simulink model "Copy_of_Five_Level"  (Simulink 8.4)
settings: Solver=ode45  StartTime=0.0  StopTime=1  RelTol=1e-3
undefined symbols (not defined in the file or in its folder): C, Cf1, Cf2, L, Lm, Lr, p, R, Rc1, Rc2, Rdc1, Rdc2, Rdc3, Rr, Tc, Ts, Uc_init
libraries: powerlib x106, simulink x3
settings Model: Creator=wangkui02  LastModifiedBy=Administrator-

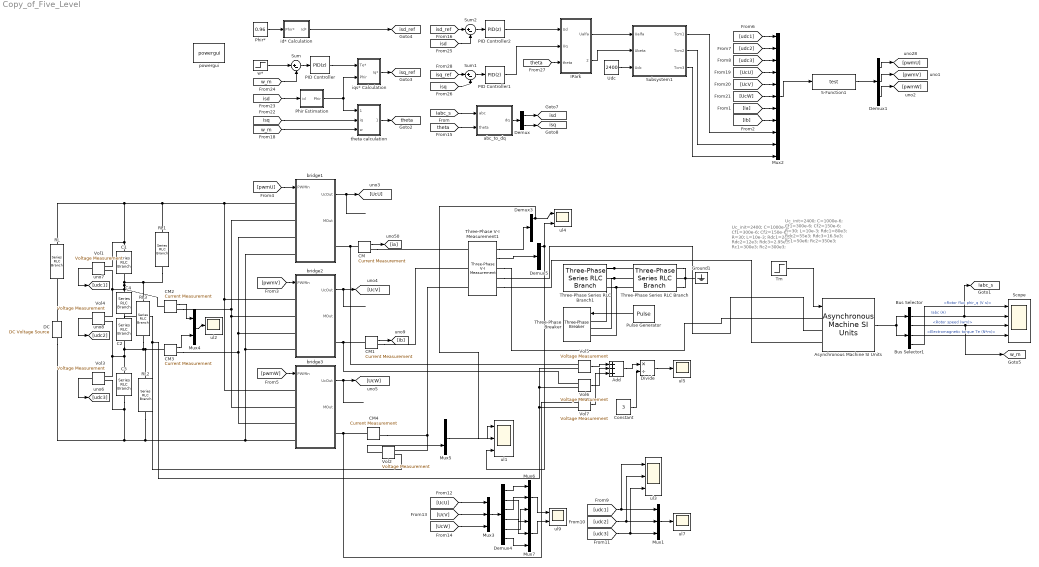
== system Copy_of_Five_Level ==
  note: Uc_init=2400;
      | C=1000e-6;
      | Cf1=300e-6;
      | Cf2=150e-6;
      | R=30;
      | L=10e-3;
      | Rdc1=2e6;
      | Rdc2=12e3;
      | Rdc3=2.95e3;
      | Rc1=300e3;
      | Rc2=300e3;
  note: Uc_init=2400;
      | C=1000e-6;
      | Cf1=300e-6;
      | Cf2=150e-6;
      | R=30;
      | L=10e-3;
      | Rdc1=80e3;
      | Rdc2=55e3;
      | Rdc3=16.5e3;
      | Rc1=50e6;
      | Rc2=350e3;
  Add : Sum  Inputs=+++
  Asynchronous Machine SI Units : powerlib/Machines/Asynchronous Machine SI Units  PresetModel=No  MechanicalLoad=Torque Tm  ShowDetailedParameters=on  RotorType=Squirrel-cage  ReferenceFrame=Stationary  Units=SI  MeasurementBus=off  NominalParameters=[2200 380 50]  Stator=[2.74 0.0138]  Rotor=[2.54 0.0138]  Cage1=[ 0.022 0.226/377]  Cage2=[ 0.022 0.226/377]  Lm=0.299  Mechanical=[0.0131 0.002985 2]  PolePairs=2  InitialConditions="[ 1,0   0,0,0   0,0,0 ]"  SimulateSaturation=off  Saturation=[14.03593122, 27.81365428, 53.79336849, 72.68890987, 97.98006896, 148.6815601, 215.7428561, 302.9841135, 428.7778367 ; 230, 322, 414, 460, 506, 552, 598, 644, 690]  LoadFlowParameters=0  TsPowergui=0  TsBlock=-1  IterativeModel=Forward Euler  Pmec=0
  Bus Selector : BusSelector  OutputSignals=Stator measurements.Stator current is_a (A),Stator measurements.Stator current is_b (A),Stator measurements.Stator current is_c (A)  OutputAsBus=on
  Bus Selector1 : BusSelector  OutputSignals=Mechanical.Rotor speed (wm),Mechanical.Electromagnetic torque Te (N*m),Rotor measurements.Rotor flux phir_q (V s)
  C1 : powerlib/Elements/Series RLC Branch  LConnTagsString=__new0  RConnTagsString=__new0  BranchType=C  Resistance=0.01  Inductance=1e-3  SetiL0=off  InitialCurrent=0  Capacitance=C  Setx0=on  InitialVoltage=Uc_init*1  Measurements=None
  C2 : powerlib/Elements/Series RLC Branch  LConnTagsString=__new0  RConnTagsString=__new0  BranchType=C  Resistance=0.01  Inductance=1e-3  SetiL0=off  InitialCurrent=0  Capacitance=C  Setx0=on  InitialVoltage=Uc_init  Measurements=None
  C3 : powerlib/Elements/Series RLC Branch  LConnTagsString=__new0  RConnTagsString=__new0  BranchType=C  Resistance=0.01  Inductance=1e-3  SetiL0=off  InitialCurrent=0  Capacitance=C*1  Setx0=on  InitialVoltage=Uc_init*1  Measurements=None
  C4 : powerlib/Elements/Series RLC Branch  LConnTagsString=__new0  RConnTagsString=__new0  BranchType=C  Resistance=0.01  Inductance=1e-3  SetiL0=off  InitialCurrent=0  Capacitance=C  Setx0=on  InitialVoltage=Uc_init  Measurements=None
  CM{,1..4} (5 alike) : powerlib/Measurements/Current Measurement  PhasorSimulation=off  OutputType=Complex  PSBequivalent=0
  Constant : Constant  Value=3
  DC : powerlib/Electrical Sources/DC Voltage Source  Amplitude=Uc_init*4  Measurements=None
  Demux : Demux  Outputs=2
  Demux1 : Demux  Outputs=[10 10 10]
  Demux3 : Demux  Outputs=3
  Demux4 : Demux  Outputs=6
  Demux5 : Demux  Outputs=3
  Divide : Product  Inputs=*/
  Ground1 : powerlib/Elements/Ground  LConnTagsString=a
  IPark : Subsystem
  Mux1 : Mux  Inputs=3
  Mux2 : Mux  Inputs=[1 1 1 2 2 2 1 1 1 1 1]
  Mux3 : Mux  Inputs=[2 2 2]
  Mux4 : Mux  Inputs=2
  Mux5 : Mux  Inputs=2
  Mux6 : Mux  Inputs=3
  Mux7 : Mux  Inputs=3
  PID Controller : simulink/Continuous/PID Controller  Controller=PID  TimeDomain=Discrete-time  SampleTime=Tc  IntegratorMethod=Forward Euler  FilterMethod=Forward Euler  Form=Parallel  P=0.075  I=10  D=0  N=100  InitialConditionSource=internal  InitialConditionForIntegrator=0  InitialConditionForFilter=0  ExternalReset=none  LimitOutput=on  UpperSaturationLimit=20  LowerSaturationLimit=-20  LinearizeAsGain=on  AntiWindupMode=none  Kb=1  TrackingMode=off  Kt=1  PParamMin=[]  PParamMax=[]  IParamMin=[]  IParamMax=[]  DParamMin=[]  DParamMax=[]  NParamMin=[]  NParamMax=[]  KbParamMin=[]  KbParamMax=[]  KtParamMin=[]  KtParamMax=[]  POutMin=[]  POutMax=[]  IOutMin=[]  IOutMax=[]  DOutMin=[]  DOutMax=[]  NOutMin=[]  NOutMax=[]  KbOutMin=[]  KbOutMax=[]  KtOutMin=[]  KtOutMax=[]  IntegratorOutMin=[]  IntegratorOutMax=[]  FilterOutMin=[]  FilterOutMax=[]  SumOutMin=[]  SumOutMax=[]  SumI1OutMin=[]  SumI1OutMax=[]  SumI2OutMin=[]  SumI2OutMax=[]  SumI3OutMin=[]  SumI3OutMax=[]  SumDOutMin=[]  SumDOutMax=[]  SaturationOutMin=[]  SaturationOutMax=[]  IntegratorContinuousStateAttributes=''  IntegratorStateMustResolveToSignalObject=off  IntegratorRTWStateStorageClass=Auto  FilterContinuousStateAttributes=''  FilterStateMustResolveToSignalObject=off  FilterRTWStateStorageClass=Auto  DifferentiatorICPrevScaledInput=0  DifferentiatorOutMin=[]  DifferentiatorOutMax=[]  UseFilter=on
  PID Controller1 : simulink/Continuous/PID Controller  Controller=PID  TimeDomain=Discrete-time  SampleTime=Tc  IntegratorMethod=Forward Euler  FilterMethod=Forward Euler  Form=Parallel  P=20  I=200  D=0  N=100  InitialConditionSource=internal  InitialConditionForIntegrator=0  InitialConditionForFilter=0  ExternalReset=none  LimitOutput=on  UpperSaturationLimit=500  LowerSaturationLimit=-500  LinearizeAsGain=on  AntiWindupMode=none  Kb=1  TrackingMode=off  Kt=1  PParamMin=[]  PParamMax=[]  IParamMin=[]  IParamMax=[]  DParamMin=[]  DParamMax=[]  NParamMin=[]  NParamMax=[]  KbParamMin=[]  KbParamMax=[]  KtParamMin=[]  KtParamMax=[]  POutMin=[]  POutMax=[]  IOutMin=[]  IOutMax=[]  DOutMin=[]  DOutMax=[]  NOutMin=[]  NOutMax=[]  KbOutMin=[]  KbOutMax=[]  KtOutMin=[]  KtOutMax=[]  IntegratorOutMin=[]  IntegratorOutMax=[]  FilterOutMin=[]  FilterOutMax=[]  SumOutMin=[]  SumOutMax=[]  SumI1OutMin=[]  SumI1OutMax=[]  SumI2OutMin=[]  SumI2OutMax=[]  SumI3OutMin=[]  SumI3OutMax=[]  SumDOutMin=[]  SumDOutMax=[]  SaturationOutMin=[]  SaturationOutMax=[]  IntegratorContinuousStateAttributes=''  IntegratorStateMustResolveToSignalObject=off  IntegratorRTWStateStorageClass=Auto  FilterContinuousStateAttributes=''  FilterStateMustResolveToSignalObject=off  FilterRTWStateStorageClass=Auto  DifferentiatorICPrevScaledInput=0  DifferentiatorOutMin=[]  DifferentiatorOutMax=[]  UseFilter=on
  PID Controller2 : simulink/Continuous/PID Controller  Controller=PID  TimeDomain=Discrete-time  SampleTime=Tc  IntegratorMethod=Forward Euler  FilterMethod=Forward Euler  Form=Parallel  P=20  I=200  D=0  N=100  InitialConditionSource=internal  InitialConditionForIntegrator=0  InitialConditionForFilter=0  ExternalReset=none  LimitOutput=on  UpperSaturationLimit=500  LowerSaturationLimit=-500  LinearizeAsGain=on  AntiWindupMode=none  Kb=1  TrackingMode=off  Kt=1  PParamMin=[]  PParamMax=[]  IParamMin=[]  IParamMax=[]  DParamMin=[]  DParamMax=[]  NParamMin=[]  NParamMax=[]  KbParamMin=[]  KbParamMax=[]  KtParamMin=[]  KtParamMax=[]  POutMin=[]  POutMax=[]  IOutMin=[]  IOutMax=[]  DOutMin=[]  DOutMax=[]  NOutMin=[]  NOutMax=[]  KbOutMin=[]  KbOutMax=[]  KtOutMin=[]  KtOutMax=[]  IntegratorOutMin=[]  IntegratorOutMax=[]  FilterOutMin=[]  FilterOutMax=[]  SumOutMin=[]  SumOutMax=[]  SumI1OutMin=[]  SumI1OutMax=[]  SumI2OutMin=[]  SumI2OutMax=[]  SumI3OutMin=[]  SumI3OutMax=[]  SumDOutMin=[]  SumDOutMax=[]  SaturationOutMin=[]  SaturationOutMax=[]  IntegratorContinuousStateAttributes=''  IntegratorStateMustResolveToSignalObject=off  IntegratorRTWStateStorageClass=Auto  FilterContinuousStateAttributes=''  FilterStateMustResolveToSignalObject=off  FilterRTWStateStorageClass=Auto  DifferentiatorICPrevScaledInput=0  DifferentiatorOutMin=[]  DifferentiatorOutMax=[]  UseFilter=on
  Phir Estimation : Subsystem
  Phir* : Constant  Value=0.96
  Pulse Generator : DiscretePulseGenerator  PulseType=Time based  PulseWidth=50
  RL : powerlib/Elements/Series RLC Branch  LConnTagsString=__new0  RConnTagsString=__new0  BranchType=RL  Resistance=0.01  Inductance=1e-6  SetiL0=off  InitialCurrent=0  Capacitance=1e-6  Setx0=off  InitialVoltage=0  Measurements=None
  RL1 : powerlib/Elements/Series RLC Branch  LConnTagsString=__new0  RConnTagsString=__new0  BranchType=R  Resistance=Rdc1  Inductance=1e-6  SetiL0=off  InitialCurrent=0  Capacitance=1e-6  Setx0=off  InitialVoltage=0  Measurements=None
  RL2 : powerlib/Elements/Series RLC Branch  LConnTagsString=__new0  RConnTagsString=__new0  BranchType=R  Resistance=Rdc3  Inductance=1e-6  SetiL0=off  InitialCurrent=0  Capacitance=1e-6  Setx0=off  InitialVoltage=0  Measurements=None
  RL3 : powerlib/Elements/Series RLC Branch  LConnTagsString=__new0  RConnTagsString=__new0  BranchType=R  Resistance=Rdc2  Inductance=1e-6  SetiL0=off  InitialCurrent=0  Capacitance=1e-6  Setx0=off  InitialVoltage=0  Measurements=None
  S-Function1 : S-Function  FunctionName=test  EnableBusSupport=off
  Scope : Scope  NumInputPorts=4
      settings: YMin=-0.1~-40~-20~-5  YMax=0.4~40~5~10  SaveName=ScopeData9  Decimation=20  SampleTime=5e-6
  Subsystem1 : Subsystem
  Sum : Sum  Inputs=|+-
  Sum1 : Sum  Inputs=|+-
  Sum2 : Sum  Inputs=|+-
  Three-Phase Series RLC Branch : powerlib/Elements/Three-Phase Series RLC Branch  LConnTagsString=A|B|C  RConnTagsString=A|B|C  BranchType=RL  Resistance=R  Inductance=L  Capacitance=1e-6  Measurements=Branch voltages and currents
  Three-Phase Series RLC Branch1 : powerlib/Elements/Three-Phase Series RLC Branch  LConnTagsString=A|B|C  RConnTagsString=A|B|C  BranchType=RL  Resistance=R  Inductance=L  Capacitance=1e-6  Measurements=Branch voltages and currents
  Three-Phase V-I Measurement1 : powerlib/Measurements/Three-Phase V-I Measurement  VoltageMeasurement=phase-to-phase  SetLabelV=off  LabelV=Vabc  Vpu=off  VpuLL=off  CurrentMeasurement=yes  SetLabelI=off  LabelI=Iabc  Ipu=off  Pbase=100e6  Vbase=500e3  OutputType=Complex  PhasorSimulation=off  PSBequivalent=0
  Three-Phase Breaker : powerlib/Elements/Three-Phase Breaker  InitialState=closed  SwitchA=on  SwitchB=on  SwitchC=on  SwitchTimes="[4/60  10/60]"  External=on  BreakerResistance=0.001  SnubberResistance=1e6  SnubberCapacitance=inf  Measurements=None
  Tm : Step  Time=0.1  After=5  SampleTime=0
  Udc : Constant  Value=2400
  Vol{1..7} (7 alike) : powerlib/Measurements/Voltage Measurement  PhasorSimulation=off  OutputType=Complex  PSBequivalent=0
  abc_to_dq : Subsystem
  bridge1 : Subsystem
  bridge2 : Subsystem
  bridge3 : Subsystem
  id* Calculation : Subsystem
  iqs* Calculation : Subsystem
  powergui : powerlib/powergui  Priority=1  SimulationMode=Discrete  SolverType=Tustin/Backward Euler (TBE)  SampleTime=Ts  frequency=60  SPID=off  DisableSnubberDevices=off  DisableRonSwitches=off  DisableVfSwitches=off  SwTol=0  DisplayEquations=off  Interpol=off  methode=off  Ts=10  frequencyindice=0  Pbase=100e6  ErrMax=1e-4  Iterations=50  UnitsV=kV  UnitsW=MW  FunctionMessages=off  echomessages=off  HookPort=off  EnableUseOfTLC=off  x0status=blocks  RestoreLinks=warning  ResistiveCurrentMeasurement=off  Frange=[0:2:500]  Ylog=off  Xlog=on  ShowGrid=off  save=off  variable=ZData  structure=0  ZoomFFT=off  StartTime=0.0  cycles=1  DisplayStyle=1  fundamental=60  FreqAxis=off  MaxFrequency=1000  frequencyindicesteady=1  RmsSteady=1  display=off
  theta calculation : Subsystem  mask{Lr=Lr, Lm=Lm, Rr=Rr}
  ul1 : Scope  NumInputPorts=3
      settings: YMin=-5000~-10000~-150  YMax=5000~10000~150  SaveName=io  MaxDataPoints=100000  Decimation=10
  ul2 : Scope
      settings: YMin=-200  YMax=200  SaveName=udc1  MaxDataPoints=100000  Decimation=10
  ul3 : Scope  NumInputPorts=3
      settings: TimeRange=1  YMin=2385~4780~2340  YMax=2405~4900~2400  SaveName=ucf1  MaxDataPoints=100000
  ul4 : Scope  NumInputPorts=2
      settings: YMin=-0.0025~-4  YMax=0.001~14  SaveName=ul  MaxDataPoints=100000  Decimation=10
  ul5 : Scope
      settings: TimeRange=1  YMin=-5000  YMax=-1500  SaveName=udc2  MaxDataPoints=100000  Decimation=10
  ul7 : Scope
      settings: YMin=2000  YMax=5000  SaveName=udc  MaxDataPoints=100000  Decimation=10
  ul9 : Scope  NumInputPorts=2
      settings: TimeRange=0.2  YMin=4500~2395  YMax=4850~2440  SaveName=ucf  MaxDataPoints=100000
  w* : Step  Time=0.01  After=1000/30*pi  SampleTime=0
  tag scope: Iabc_s=global, isd=global, isd_ref=global, isq=global, isq_ref=global, theta=global, w_m=global
  wires:
  bridge1/1(UcOut) -> [UcU]
  [pwmU] -> bridge1/1(PWMIn)
  [pwmV] -> bridge2/1(PWMIn)
  [pwmW] -> bridge3/1(PWMIn)
  Vol2/1 -> Mux5/2
  bridge2/1(UcOut) -> [UcV]
  Vol1/1 -> [udc1]
  Vol3/1 -> [udc3]
  bridge3/1(UcOut) -> [UcW]
  Vol4/1 -> [udc2]
  [udc1] -> Mux1/1, ul3/1
  [udc2] -> Mux1/2, ul3/2
  [udc3] -> Mux1/3, ul3/3
  Mux1/1 -> ul7/1
  Three-Phase V-I Measurement1/1 -> Demux3/1
  Demux3/1 -> ul4/1, ul1/2
  CM/1 -> [ia]
  CM1/1 -> [ib]
  [UcU] -> Mux3/1
  [UcV] -> Mux3/2
  [UcW] -> Mux3/3
  Pulse Generator/1 -> Three-Phase Breaker/1
  CM2/1 -> Mux4/1
  Mux4/1 -> ul2/1
  CM3/1 -> Mux4/2
  Mux5/1 -> ul1/1
  Mux3/1 -> Demux4/1
  Demux4/1 -> Mux6/1
  Demux4/3 -> Mux6/2
  Demux4/5 -> Mux6/3
  Demux4/2 -> Mux7/1
  Demux4/4 -> Mux7/2
  Mux6/1 -> ul9/1
  Mux7/1 -> ul9/2
  Demux4/6 -> Mux7/3
  Three-Phase V-I Measurement1/2 -> Demux5/1
  Demux5/1 -> ul4/2, ul1/3
  Vol5/1 -> Add/1
  Vol6/1 -> Add/2
  Vol7/1 -> Add/3
  Divide/1 -> ul5/1
  Add/1 -> Divide/1
  Constant/1 -> Divide/2
  [Iabc_s] -> abc_to_dq/1(abc)
  [theta] -> abc_to_dq/2(theta)
  abc_to_dq/1(dq) -> Demux/1
  Demux/1 -> [isd]
  Demux/2 -> [isq]
  Phir*/1 -> id* Calculation/1(Phir*)
  PID Controller/1 -> iqs* Calculation/1(Te*)
  [w_m] -> theta calculation/3(w)
  Phir Estimation/1(Phir) -> theta calculation/1(Phir), iqs* Calculation/2(Phir)
  [isq] -> theta calculation/2(iq)
  [isd] -> Phir Estimation/1(id)
  [w_m] -> Sum/2
  theta calculation/1(theta) -> [theta]
  [isd] -> Sum2/2
  PID Controller1/1 -> IPark/2(Uq)
  [theta] -> IPark/3(theta)
  Sum/1 -> PID Controller/1
  w*/1 -> Sum/1
  iqs* Calculation/1(Iq*) -> [isq_ref]
  Sum1/1 -> PID Controller1/1
  [isq_ref] -> Sum1/1
  [isq] -> Sum1/2
  id* Calculation/1(Id*) -> [isd_ref]
  [isd_ref] -> Sum2/1
  Sum2/1 -> PID Controller2/1
  PID Controller2/1 -> IPark/1(Ud)
  Udc/1 -> Subsystem1/3(Udc)
  IPark/1(Ualfa) -> Subsystem1/1(Ualfa)
  IPark/2(Ubeta) -> Subsystem1/2(Ubeta)
  Tm/1 -> Asynchronous Machine SI Units/1
  Subsystem1/1(Tcm1) -> Mux2/9
  Demux1/1 -> [pwmU]
  Demux1/2 -> [pwmV]
  Demux1/3 -> [pwmW]
  [udc1] -> Mux2/1
  [udc2] -> Mux2/2
  [UcU] -> Mux2/4
  [UcV] -> Mux2/5
  [UcW] -> Mux2/6
  [ia] -> Mux2/7
  [ib] -> Mux2/8
  [udc3] -> Mux2/3
  Subsystem1/2(Tcm2) -> Mux2/10
  Subsystem1/3(Tcm3) -> Mux2/11
  Bus Selector1/1 -> Scope/3, [w_m]  "<Rotor speed (wm)>"
  Bus Selector/1 -> [Iabc_s], Scope/2  "Iabc (A)"
  Bus Selector1/2 -> Scope/4  "<Electromagnetic torque Te (N*m)>"
  Asynchronous Machine SI Units/1 -> Bus Selector/1, Bus Selector1/1
  Bus Selector1/3 -> Scope/1  "<Rotor flux phir_q (V s)>"
  Mux2/1 -> S-Function1/1
  S-Function1/1 -> Demux1/1
  connections:
  Ground1/LConn1 -- Three-Phase Series RLC Branch/RConn2 -- Three-Phase Series RLC Branch/RConn1 -- Three-Phase Series RLC Branch/RConn3
  Three-Phase V-I Measurement1/LConn3 -- Vol2/LConn1 -- CM4/RConn1
  C1/LConn1 -- Vol1/LConn1 -- RL/LConn1 -- bridge3/LConn1 -- bridge2/LConn1 -- bridge1/LConn1 -- RL1/LConn1
  C3/RConn1 -- Vol3/LConn2 -- DC/LConn1 -- bridge3/LConn4 -- bridge1/LConn4 -- bridge2/LConn4 -- RL2/RConn1
  DC/RConn1 -- RL/RConn1
  bridge3/LConn3 -- bridge1/LConn3 -- bridge2/LConn3 -- CM3/RConn1
  CM2/RConn1 -- bridge3/LConn2 -- bridge2/LConn2 -- bridge1/LConn2
  CM/LConn1 -- Vol5/LConn1 -- bridge1/RConn1
  CM/RConn1 -- Three-Phase V-I Measurement1/LConn1
  bridge2/RConn1 -- Vol6/LConn1 -- CM1/LConn1
  CM1/RConn1 -- Three-Phase V-I Measurement1/LConn2
  Three-Phase V-I Measurement1/RConn1 -- Asynchronous Machine SI Units/LConn1
  Three-Phase Series RLC Branch1/RConn1 -- Three-Phase Breaker/LConn1 -- Three-Phase Series RLC Branch/LConn1
  Three-Phase Series RLC Branch1/RConn2 -- Three-Phase Breaker/LConn2 -- Three-Phase Series RLC Branch/LConn2
  Three-Phase Series RLC Branch1/RConn3 -- Three-Phase Series RLC Branch/LConn3 -- Three-Phase Breaker/LConn3
  RL1/RConn1 -- CM2/LConn1 -- Vol4/LConn1 -- Vol1/LConn2 -- C4/LConn1 -- C1/RConn1 -- RL3/LConn1
  CM3/LConn1 -- Vol4/LConn2 -- Vol3/LConn1 -- C3/LConn1 -- C2/RConn1 -- RL3/RConn1 -- RL2/LConn1
  CM4/LConn1 -- Vol7/LConn1 -- bridge3/RConn1
  C4/RConn1 -- Vol7/LConn2 -- Vol6/LConn2 -- Vol5/LConn2 -- Vol2/LConn2
  Three-Phase V-I Measurement1/RConn2 -- Asynchronous Machine SI Units/LConn2
  Three-Phase V-I Measurement1/RConn3 -- Asynchronous Machine SI Units/LConn3

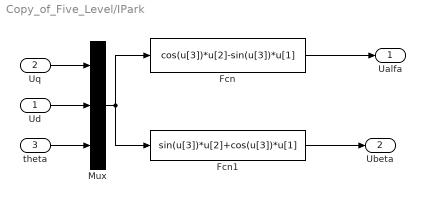
== system Copy_of_Five_Level/IPark ==
  Ud : Inport
  Uq : Inport  Port=2
  theta : Inport  Port=3
  Fcn : Fcn  Expr=cos(u[3])*u[2]-sin(u[3])*u[1]
  Fcn1 : Fcn  Expr=sin(u[3])*u[2]+cos(u[3])*u[1]
  Mux : Mux  Inputs=3
  Ualfa : Outport
  Ubeta : Outport  Port=2
  wires:
  Uq/1 -> Mux/1
  Ud/1 -> Mux/2
  theta/1 -> Mux/3
  Mux/1 -> Fcn/1, Fcn1/1
  Fcn/1 -> Ualfa/1
  Fcn1/1 -> Ubeta/1

== system Copy_of_Five_Level/Phir Estimation ==
  id : Inport
  Gain : Gain  Gain=Lm*Rr  SaturateOnIntegerOverflow=on  OutDataTypeStr=Inherit: Same as input  ParamDataTypeStr=Inherit: Same as input
  Transfer Fcn : TransferFcn  Denominator=[Lr Rr]
  Phir : Outport
  wires:
  Transfer Fcn/1 -> Phir/1
  Gain/1 -> Transfer Fcn/1
  id/1 -> Gain/1

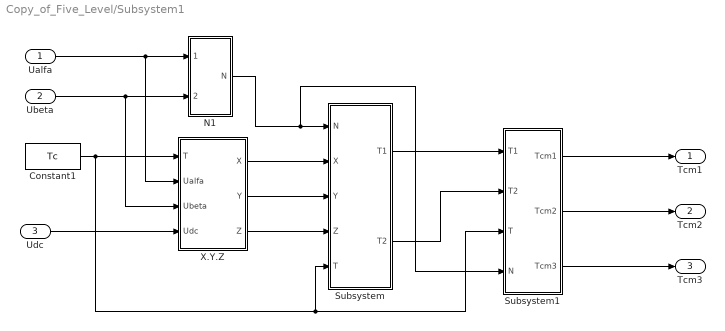
== system Copy_of_Five_Level/Subsystem1 ==
  Ualfa : Inport
  Ubeta : Inport  Port=2
  Udc : Inport  Port=3
  Constant1 : Constant  Value=Tc
  N1 : Subsystem
  Subsystem : Subsystem
  Subsystem1 : Subsystem
  X.Y.Z : Subsystem
  Tcm1 : Outport
  Tcm2 : Outport  Port=2
  Tcm3 : Outport  Port=3
  wires:
  Constant1/1 -> Subsystem1/3(T), Subsystem/5(T), X.Y.Z/1(T)
  X.Y.Z/1(X) -> Subsystem/2(X)
  X.Y.Z/2(Y) -> Subsystem/3(Y)
  X.Y.Z/3(Z) -> Subsystem/4(Z)
  Subsystem1/1(Tcm1) -> Tcm1/1
  Subsystem1/2(Tcm2) -> Tcm2/1
  Subsystem1/3(Tcm3) -> Tcm3/1
  Subsystem/1(T1) -> Subsystem1/1(T1)
  Subsystem/2(T2) -> Subsystem1/2(T2)
  N1/1(N) -> Subsystem/1(N), Subsystem1/4(N)
  Udc/1 -> X.Y.Z/4(Udc)
  Ualfa/1 -> X.Y.Z/2(Ualfa), N1/1(Ualfa)
  Ubeta/1 -> X.Y.Z/3(Ubeta), N1/2(Ubeta)

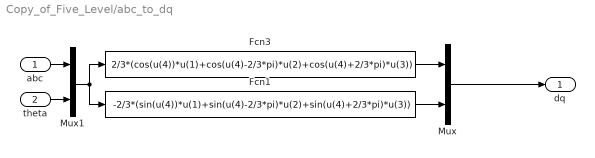
== system Copy_of_Five_Level/abc_to_dq ==
  abc : Inport
  theta : Inport  Port=2
  Fcn1 : Fcn  Expr=-2/3*(sin(u(4))*u(1)+sin(u(4)-2/3*pi)*u(2)+sin(u(4)+2/3*pi)*u(3))
  Fcn3 : Fcn  Expr=2/3*(cos(u(4))*u(1)+cos(u(4)-2/3*pi)*u(2)+cos(u(4)+2/3*pi)*u(3))
  Mux : Mux  Inputs=2
  Mux1 : Mux  Inputs=2
  dq : Outport
  wires:
  Fcn3/1 -> Mux/1
  Fcn1/1 -> Mux/2
  abc/1 -> Mux1/1
  theta/1 -> Mux1/2
  Mux1/1 -> Fcn3/1, Fcn1/1
  Mux/1 -> dq/1

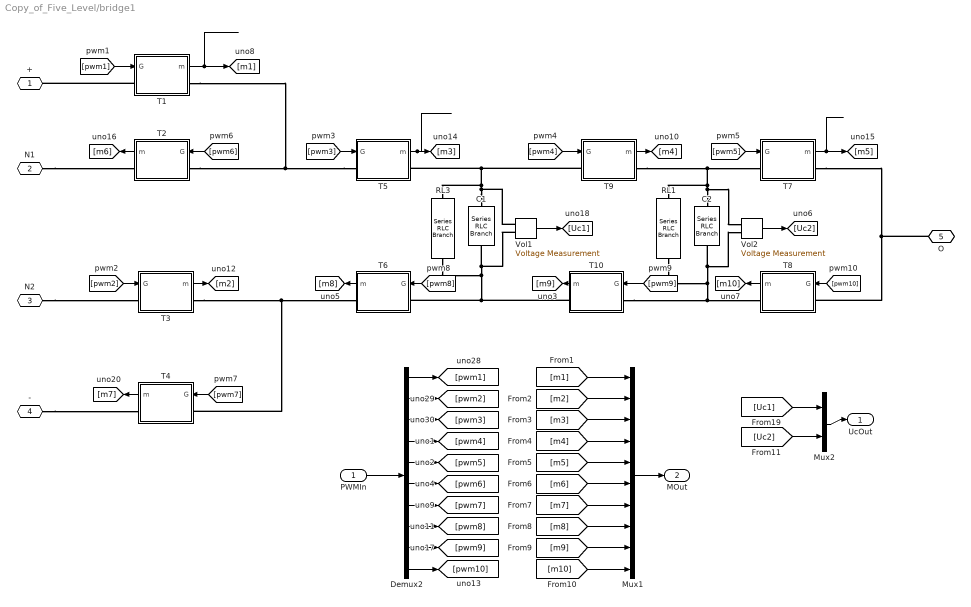
== system Copy_of_Five_Level/bridge1 ==
  PWMIn : Inport
  C1 : powerlib/Elements/Series RLC Branch  LConnTagsString=__new0  RConnTagsString=__new0  BranchType=C  Resistance=1  Inductance=1e-3  SetiL0=off  InitialCurrent=0  Capacitance=Cf2  Setx0=on  InitialVoltage=Uc_init*2*1  Measurements=None
  C2 : powerlib/Elements/Series RLC Branch  LConnTagsString=__new0  RConnTagsString=__new0  BranchType=C  Resistance=1  Inductance=1e-3  SetiL0=off  InitialCurrent=0  Capacitance=Cf1  Setx0=on  InitialVoltage=Uc_init*1  Measurements=None
  Demux2 : Demux  Outputs=10
  Mux1 : Mux  Inputs=10
  Mux2 : Mux  Inputs=2
  RL1 : powerlib/Elements/Series RLC Branch  LConnTagsString=__new0  RConnTagsString=__new0  BranchType=R  Resistance=Rc1  Inductance=1e-6  SetiL0=off  InitialCurrent=0  Capacitance=1e-6  Setx0=off  InitialVoltage=0  Measurements=None
  RL3 : powerlib/Elements/Series RLC Branch  LConnTagsString=__new0  RConnTagsString=__new0  BranchType=R  Resistance=Rc2  Inductance=1e-6  SetiL0=off  InitialCurrent=0  Capacitance=1e-6  Setx0=off  InitialVoltage=0  Measurements=None
  T1 : Subsystem
  T10 : Subsystem
  T2 : Subsystem
  T3 : Subsystem
  T4 : Subsystem
  T5 : Subsystem
  T6 : Subsystem
  T7 : Subsystem
  T8 : Subsystem
  T9 : Subsystem
  Vol1 : powerlib/Measurements/Voltage Measurement  PhasorSimulation=off  OutputType=Complex  PSBequivalent=0
  Vol2 : powerlib/Measurements/Voltage Measurement  PhasorSimulation=off  OutputType=Complex  PSBequivalent=0
  + : PMIOPort  Port=1  Side=Left
  N1 : PMIOPort  Port=2  Side=Left
  N2 : PMIOPort  Port=3  Side=Left
  - : PMIOPort  Port=4  Side=Left
  O : PMIOPort  Port=5  Side=Right
  UcOut : Outport
  MOut : Outport  Port=2
  wires:
  T1/1(m) -> [m1]
  [pwm2] -> T3/1(G)
  T3/1(m) -> [m2]
  [pwm3] -> T5/1(G)
  T5/1(m) -> [m3]
  [pwm5] -> T7/1(G)
  T7/1(m) -> [m5]
  [pwm6] -> T2/1(G)
  [pwm7] -> T4/1(G)
  T4/1(m) -> [m7]
  PWMIn/1 -> Demux2/1
  Demux2/1 -> [pwm1]
  Demux2/2 -> [pwm2]
  Demux2/3 -> [pwm3]
  Demux2/4 -> [pwm4]
  Demux2/5 -> [pwm5]
  Demux2/6 -> [pwm6]
  Demux2/7 -> [pwm7]
  Demux2/8 -> [pwm8]
  [pwm1] -> T1/1(G)
  T2/1(m) -> [m6]
  [m1] -> Mux1/1
  [m2] -> Mux1/2
  [m3] -> Mux1/3
  [m4] -> Mux1/4
  [m5] -> Mux1/5
  [m6] -> Mux1/6
  [m7] -> Mux1/7
  [m8] -> Mux1/8
  Mux1/1 -> MOut/1
  [pwm10] -> T8/1(G)
  T8/1(m) -> [m10]
  [pwm8] -> T6/1(G)
  T6/1(m) -> [m8]
  Vol2/1 -> [Uc2]
  [pwm4] -> T9/1(G)
  [pwm9] -> T10/1(G)
  T10/1(m) -> [m9]
  T9/1(m) -> [m4]
  Demux2/9 -> [pwm9]
  Demux2/10 -> [pwm10]
  [m9] -> Mux1/9
  [m10] -> Mux1/10
  Vol1/1 -> [Uc1]
  Mux2/1 -> UcOut/1
  [Uc1] -> Mux2/1
  [Uc2] -> Mux2/2
  connections:
  T1/LConn1 -- +/RConn1
  -/RConn1 -- T4/RConn1
  C2/RConn1 -- Vol2/LConn2 -- T10/LConn1 -- T8/RConn1 -- RL1/RConn1
  C2/LConn1 -- Vol2/LConn1 -- T7/LConn1 -- T9/RConn1 -- RL1/LConn1
  T8/LConn1 -- O/RConn1 -- T7/RConn1
  N1/RConn1 -- T2/RConn1
  N2/RConn1 -- T3/LConn1
  T5/LConn1 -- T1/RConn1 -- T2/LConn1
  T3/RConn1 -- T6/RConn1 -- T4/LConn1
  C1/RConn1 -- Vol1/LConn2 -- T10/RConn1 -- T6/LConn1 -- RL3/RConn1
  C1/LConn1 -- T9/LConn1 -- T5/RConn1 -- RL3/LConn1 -- Vol1/LConn1

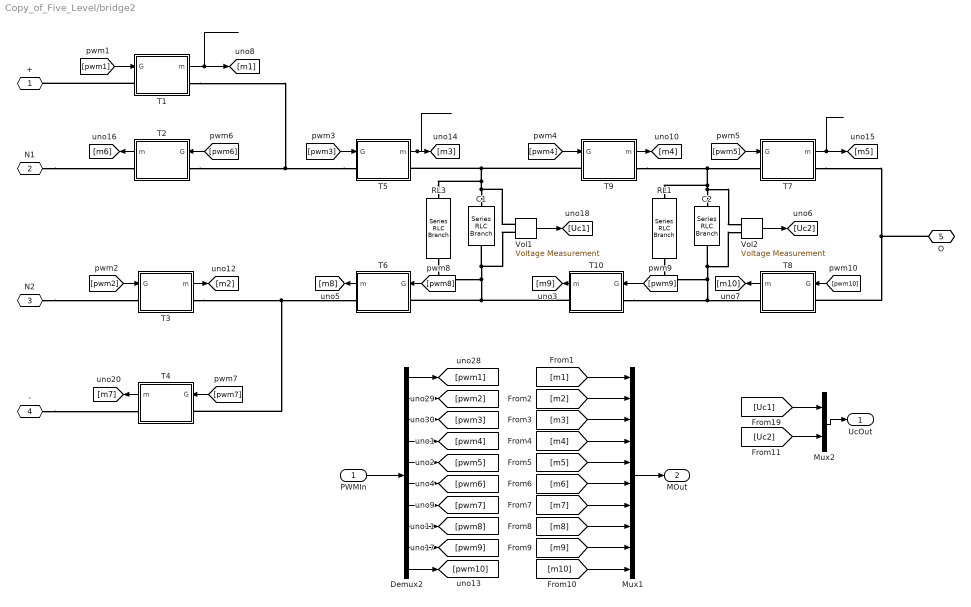
== system Copy_of_Five_Level/bridge2 ==
  PWMIn : Inport
  C1 : powerlib/Elements/Series RLC Branch  LConnTagsString=__new0  RConnTagsString=__new0  BranchType=C  Resistance=1  Inductance=1e-3  SetiL0=off  InitialCurrent=0  Capacitance=Cf2  Setx0=on  InitialVoltage=Uc_init*2  Measurements=None
  C2 : powerlib/Elements/Series RLC Branch  LConnTagsString=__new0  RConnTagsString=__new0  BranchType=C  Resistance=1  Inductance=1e-3  SetiL0=off  InitialCurrent=0  Capacitance=Cf1  Setx0=on  InitialVoltage=Uc_init  Measurements=None
  Demux2 : Demux  Outputs=10
  Mux1 : Mux  Inputs=10
  Mux2 : Mux  Inputs=2
  RL1 : powerlib/Elements/Series RLC Branch  LConnTagsString=__new0  RConnTagsString=__new0  BranchType=R  Resistance=Rc1  Inductance=1e-6  SetiL0=off  InitialCurrent=0  Capacitance=1e-6  Setx0=off  InitialVoltage=0  Measurements=None
  RL3 : powerlib/Elements/Series RLC Branch  LConnTagsString=__new0  RConnTagsString=__new0  BranchType=R  Resistance=Rc2  Inductance=1e-6  SetiL0=off  InitialCurrent=0  Capacitance=1e-6  Setx0=off  InitialVoltage=0  Measurements=None
  T1 : Subsystem
  T10 : Subsystem
  T2 : Subsystem
  T3 : Subsystem
  T4 : Subsystem
  T5 : Subsystem
  T6 : Subsystem
  T7 : Subsystem
  T8 : Subsystem
  T9 : Subsystem
  Vol1 : powerlib/Measurements/Voltage Measurement  PhasorSimulation=off  OutputType=Complex  PSBequivalent=0
  Vol2 : powerlib/Measurements/Voltage Measurement  PhasorSimulation=off  OutputType=Complex  PSBequivalent=0
  + : PMIOPort  Port=1  Side=Left
  N1 : PMIOPort  Port=2  Side=Left
  N2 : PMIOPort  Port=3  Side=Left
  - : PMIOPort  Port=4  Side=Left
  O : PMIOPort  Port=5  Side=Right
  UcOut : Outport
  MOut : Outport  Port=2
  wires:
  T1/1(m) -> [m1]
  [pwm2] -> T3/1(G)
  T3/1(m) -> [m2]
  [pwm3] -> T5/1(G)
  T5/1(m) -> [m3]
  [pwm5] -> T7/1(G)
  T7/1(m) -> [m5]
  [pwm6] -> T2/1(G)
  [pwm7] -> T4/1(G)
  T4/1(m) -> [m7]
  PWMIn/1 -> Demux2/1
  Demux2/1 -> [pwm1]
  Demux2/2 -> [pwm2]
  Demux2/3 -> [pwm3]
  Demux2/4 -> [pwm4]
  Demux2/5 -> [pwm5]
  Demux2/6 -> [pwm6]
  Demux2/7 -> [pwm7]
  Demux2/8 -> [pwm8]
  [pwm1] -> T1/1(G)
  T2/1(m) -> [m6]
  [m1] -> Mux1/1
  [m2] -> Mux1/2
  [m3] -> Mux1/3
  [m4] -> Mux1/4
  [m5] -> Mux1/5
  [m6] -> Mux1/6
  [m7] -> Mux1/7
  [m8] -> Mux1/8
  Mux1/1 -> MOut/1
  [pwm10] -> T8/1(G)
  T8/1(m) -> [m10]
  [pwm8] -> T6/1(G)
  T6/1(m) -> [m8]
  Vol2/1 -> [Uc2]
  [pwm4] -> T9/1(G)
  [pwm9] -> T10/1(G)
  T10/1(m) -> [m9]
  T9/1(m) -> [m4]
  Demux2/9 -> [pwm9]
  Demux2/10 -> [pwm10]
  [m9] -> Mux1/9
  [m10] -> Mux1/10
  Vol1/1 -> [Uc1]
  Mux2/1 -> UcOut/1
  [Uc1] -> Mux2/1
  [Uc2] -> Mux2/2
  connections:
  T1/LConn1 -- +/RConn1
  -/RConn1 -- T4/RConn1
  C2/RConn1 -- Vol2/LConn2 -- T10/LConn1 -- T8/RConn1 -- RL1/RConn1
  C2/LConn1 -- Vol2/LConn1 -- T7/LConn1 -- T9/RConn1 -- RL1/LConn1
  T8/LConn1 -- O/RConn1 -- T7/RConn1
  N1/RConn1 -- T2/RConn1
  N2/RConn1 -- T3/LConn1
  T5/LConn1 -- T1/RConn1 -- T2/LConn1
  T3/RConn1 -- T6/RConn1 -- T4/LConn1
  RL3/RConn1 -- C1/RConn1 -- Vol1/LConn2 -- T10/RConn1 -- T6/LConn1
  RL3/LConn1 -- C1/LConn1 -- Vol1/LConn1 -- T9/LConn1 -- T5/RConn1

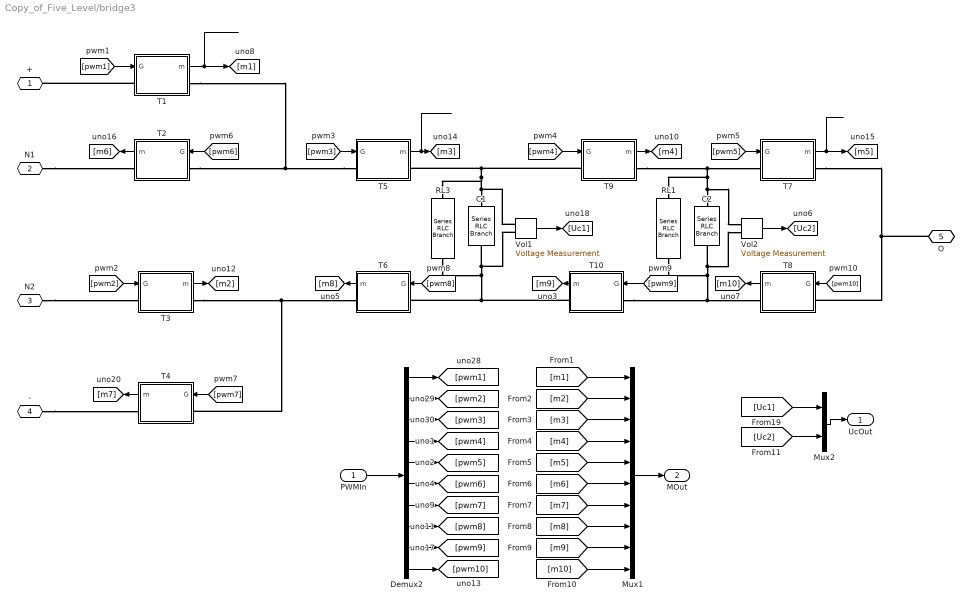
== system Copy_of_Five_Level/bridge3 ==
  PWMIn : Inport
  C1 : powerlib/Elements/Series RLC Branch  LConnTagsString=__new0  RConnTagsString=__new0  BranchType=C  Resistance=1  Inductance=1e-3  SetiL0=off  InitialCurrent=0  Capacitance=Cf2  Setx0=on  InitialVoltage=Uc_init*2*1  Measurements=None
  C2 : powerlib/Elements/Series RLC Branch  LConnTagsString=__new0  RConnTagsString=__new0  BranchType=C  Resistance=1  Inductance=1e-3  SetiL0=off  InitialCurrent=0  Capacitance=Cf1  Setx0=on  InitialVoltage=Uc_init*1  Measurements=None
  Demux2 : Demux  Outputs=10
  Mux1 : Mux  Inputs=10
  Mux2 : Mux  Inputs=2
  RL1 : powerlib/Elements/Series RLC Branch  LConnTagsString=__new0  RConnTagsString=__new0  BranchType=R  Resistance=Rc1  Inductance=1e-6  SetiL0=off  InitialCurrent=0  Capacitance=1e-6  Setx0=off  InitialVoltage=0  Measurements=None
  RL3 : powerlib/Elements/Series RLC Branch  LConnTagsString=__new0  RConnTagsString=__new0  BranchType=R  Resistance=Rc2  Inductance=1e-6  SetiL0=off  InitialCurrent=0  Capacitance=1e-6  Setx0=off  InitialVoltage=0  Measurements=None
  T1 : Subsystem
  T10 : Subsystem
  T2 : Subsystem
  T3 : Subsystem
  T4 : Subsystem
  T5 : Subsystem
  T6 : Subsystem
  T7 : Subsystem
  T8 : Subsystem
  T9 : Subsystem
  Vol1 : powerlib/Measurements/Voltage Measurement  PhasorSimulation=off  OutputType=Complex  PSBequivalent=0
  Vol2 : powerlib/Measurements/Voltage Measurement  PhasorSimulation=off  OutputType=Complex  PSBequivalent=0
  + : PMIOPort  Port=1  Side=Left
  N1 : PMIOPort  Port=2  Side=Left
  N2 : PMIOPort  Port=3  Side=Left
  - : PMIOPort  Port=4  Side=Left
  O : PMIOPort  Port=5  Side=Right
  UcOut : Outport
  MOut : Outport  Port=2
  wires:
  T1/1(m) -> [m1]
  [pwm2] -> T3/1(G)
  T3/1(m) -> [m2]
  [pwm3] -> T5/1(G)
  T5/1(m) -> [m3]
  [pwm5] -> T7/1(G)
  T7/1(m) -> [m5]
  [pwm6] -> T2/1(G)
  [pwm7] -> T4/1(G)
  T4/1(m) -> [m7]
  PWMIn/1 -> Demux2/1
  Demux2/1 -> [pwm1]
  Demux2/2 -> [pwm2]
  Demux2/3 -> [pwm3]
  Demux2/4 -> [pwm4]
  Demux2/5 -> [pwm5]
  Demux2/6 -> [pwm6]
  Demux2/7 -> [pwm7]
  Demux2/8 -> [pwm8]
  [pwm1] -> T1/1(G)
  T2/1(m) -> [m6]
  [m1] -> Mux1/1
  [m2] -> Mux1/2
  [m3] -> Mux1/3
  [m4] -> Mux1/4
  [m5] -> Mux1/5
  [m6] -> Mux1/6
  [m7] -> Mux1/7
  [m8] -> Mux1/8
  Mux1/1 -> MOut/1
  [pwm10] -> T8/1(G)
  T8/1(m) -> [m10]
  [pwm8] -> T6/1(G)
  T6/1(m) -> [m8]
  Vol2/1 -> [Uc2]
  [pwm4] -> T9/1(G)
  [pwm9] -> T10/1(G)
  T10/1(m) -> [m9]
  T9/1(m) -> [m4]
  Demux2/9 -> [pwm9]
  Demux2/10 -> [pwm10]
  [m9] -> Mux1/9
  [m10] -> Mux1/10
  Vol1/1 -> [Uc1]
  Mux2/1 -> UcOut/1
  [Uc1] -> Mux2/1
  [Uc2] -> Mux2/2
  connections:
  T1/LConn1 -- +/RConn1
  -/RConn1 -- T4/RConn1
  C2/RConn1 -- Vol2/LConn2 -- T10/LConn1 -- T8/RConn1 -- RL1/RConn1
  C2/LConn1 -- Vol2/LConn1 -- T7/LConn1 -- T9/RConn1 -- RL1/LConn1
  T8/LConn1 -- O/RConn1 -- T7/RConn1
  N1/RConn1 -- T2/RConn1
  N2/RConn1 -- T3/LConn1
  T5/LConn1 -- T1/RConn1 -- T2/LConn1
  T3/RConn1 -- T6/RConn1 -- T4/LConn1
  RL3/RConn1 -- C1/RConn1 -- Vol1/LConn2 -- T10/RConn1 -- T6/LConn1
  RL3/LConn1 -- C1/LConn1 -- Vol1/LConn1 -- T9/LConn1 -- T5/RConn1

== system Copy_of_Five_Level/id* Calculation ==
  note: Id* = Phir*/ Lm
  Phir* : Inport
  KF : Gain  Gain=1/Lm  SaturateOnIntegerOverflow=on  OutDataTypeStr=Inherit: Same as input  ParamDataTypeStr=Inherit: Same as input
  Id* : Outport
  wires:
  KF/1 -> Id*/1
  Phir*/1 -> KF/1

== system Copy_of_Five_Level/iqs* Calculation ==
  note: Iq= ( 2/3) * (2/p) * ( Lr/Lm) * (Te / Phir)
  note: Lm = 34.7 mH
  note: Lr = Ll'r +Lm = 0.8 +34.7= 35.5 mH
  note: p= nb of poles = 4
  note: Iq= 0.341 * (Te / Phir)
  Te* : Inport
  Phir : Inport  Port=2
  Fcn : Fcn  Expr=u(1)/(u(2)*Lr/Lm/p+0.00000001)
  Mux1 : Mux  Inputs=2
  Iq* : Outport  InitialOutput=0
  wires:
  Phir/1 -> Mux1/2
  Fcn/1 -> Iq*/1
  Te*/1 -> Mux1/1
  Mux1/1 -> Fcn/1

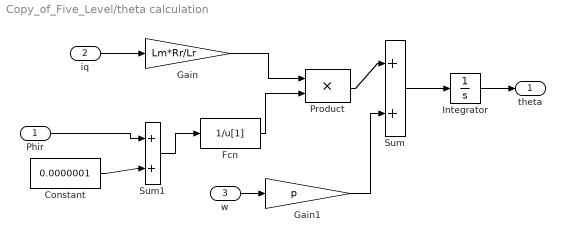
== system Copy_of_Five_Level/theta calculation ==
  Phir : Inport
  iq : Inport  Port=2
  w : Inport  Port=3
  Constant : Constant  Value=0.0000001
  Fcn : Fcn  Expr=1/u[1]
  Gain : Gain  Gain=Lm*Rr/Lr  SaturateOnIntegerOverflow=on  OutDataTypeStr=Inherit: Same as input  ParamDataTypeStr=Inherit: Same as input
  Gain1 : Gain  Gain=p  SaturateOnIntegerOverflow=on  OutDataTypeStr=Inherit: Same as input  ParamDataTypeStr=Inherit: Same as input
  Integrator : Integrator
  Product : Product  SaturateOnIntegerOverflow=on  OutDataTypeStr=Inherit: Same as first input
  Sum : Sum  Inputs=|++  SaturateOnIntegerOverflow=on
  Sum1 : Sum  Inputs=|++  SaturateOnIntegerOverflow=on
  theta : Outport
  wires:
  Product/1 -> Sum/1
  Fcn/1 -> Product/2
  Gain/1 -> Product/1
  iq/1 -> Gain/1
  Sum/1 -> Integrator/1
  Integrator/1 -> theta/1
  w/1 -> Gain1/1
  Constant/1 -> Sum1/2
  Phir/1 -> Sum1/1
  Sum1/1 -> Fcn/1
  Gain1/1 -> Sum/2

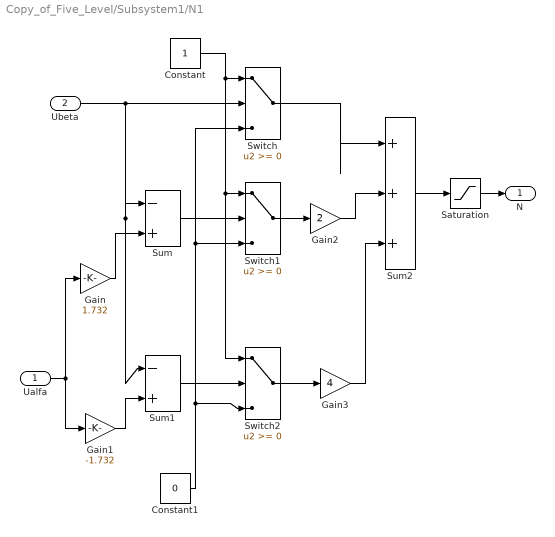
== system Copy_of_Five_Level/Subsystem1/N1 ==
  Ualfa : Inport
  Ubeta : Inport  Port=2
  Constant : Constant
  Constant1 : Constant  Value=0
  Gain : Gain  Gain=1.732
  Gain1 : Gain  Gain=-1.732
  Gain2 : Gain  Gain=2
  Gain3 : Gain  Gain=4
  Saturation : Saturate  UpperLimit=6  LowerLimit=1
  Sum : Sum  Inputs=|-+
  Sum1 : Sum  Inputs=|-+
  Sum2 : Sum  Inputs=|+++
  Switch : Switch
  Switch1 : Switch
  Switch2 : Switch
  N : Outport
  wires:
  Ubeta/1 -> Switch/2, Sum/1, Sum1/1
  Constant/1 -> Switch/1, Switch2/1, Switch1/1
  Ualfa/1 -> Gain1/1, Gain/1
  Gain/1 -> Sum/2
  Sum/1 -> Switch1/2
  Sum1/1 -> Switch2/2
  Gain1/1 -> Sum1/2
  Constant1/1 -> Switch/3, Switch1/3, Switch2/3
  Switch1/1 -> Gain2/1
  Switch2/1 -> Gain3/1
  Switch/1 -> Sum2/1
  Gain3/1 -> Sum2/3
  Gain2/1 -> Sum2/2
  Sum2/1 -> Saturation/1
  Saturation/1 -> N/1

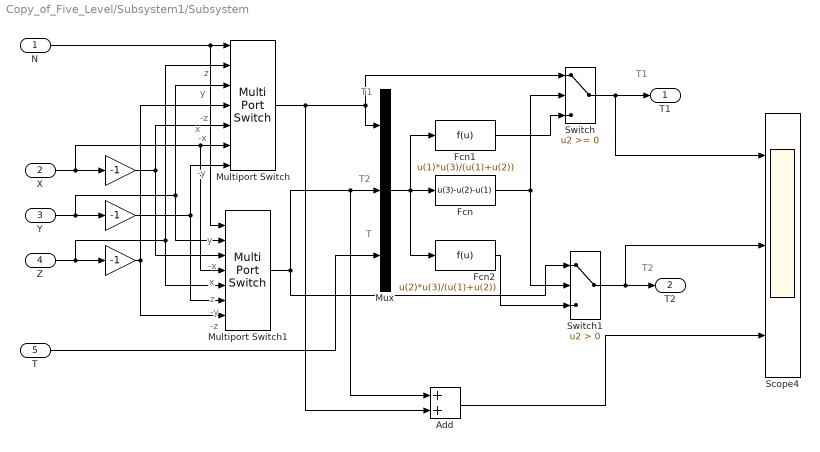
== system Copy_of_Five_Level/Subsystem1/Subsystem ==
  note: z
  note: y
  note: -z
  note: -x
  note: x
  note: -y
  note: y
  note: -x
  note: x
  note: z
  note: -y
  note: -z
  note: T1
  note: T2
  note: T
  note: T1
  note: T2
  N : Inport
  X : Inport  Port=2
  Y : Inport  Port=3
  Z : Inport  Port=4
  T : Inport  Port=5
  " " : Gain  Gain=-1
  "  " : Gain  Gain=-1
  "    " : Gain  Gain=-1
  Add : Sum
  Fcn : Fcn  Expr=u(3)-u(2)-u(1)
  Fcn1 : Fcn  Expr=u(1)*u(3)/(u(1)+u(2))
  Fcn2 : Fcn  Expr=u(2)*u(3)/(u(1)+u(2))
  Multiport Switch : MultiPortSwitch  Inputs=6
  Multiport Switch1 : MultiPortSwitch  Inputs=6
  Mux : Mux  Inputs=3
  Scope4 : Scope  NumInputPorts=3
      settings: TimeRange=0.35  YMin=-1e-005~-1e-005~0.00011  YMax=0.00018~0.00018~0.000205  SaveName=ScopeData4
  Switch : Switch
  Switch1 : Switch  Criteria=u2 > Threshold
  T1 : Outport
  T2 : Outport  Port=2
  wires:
  N/1 -> Multiport Switch1/1, Multiport Switch/1
  X/1 -> Multiport Switch1/4, Multiport Switch/6, " "/1
  Y/1 -> Multiport Switch1/2, Multiport Switch/3, "  "/1
  Z/1 -> Multiport Switch1/5, Multiport Switch/2, "    "/1
  "    "/1 -> Multiport Switch1/7, Multiport Switch/4
  "  "/1 -> Multiport Switch/7, Multiport Switch1/6
  " "/1 -> Multiport Switch/5, Multiport Switch1/3
  Multiport Switch/1 -> Mux/1, Switch/1, Add/2
  Multiport Switch1/1 -> Switch1/1, Mux/2, Add/1
  T/1 -> Mux/3
  Mux/1 -> Fcn/1, Fcn1/1, Fcn2/1
  Fcn/1 -> Switch/2, Switch1/2
  Fcn1/1 -> Switch/3
  Fcn2/1 -> Switch1/3
  Switch/1 -> T1/1, Scope4/1
  Switch1/1 -> T2/1, Scope4/2
  Add/1 -> Scope4/3

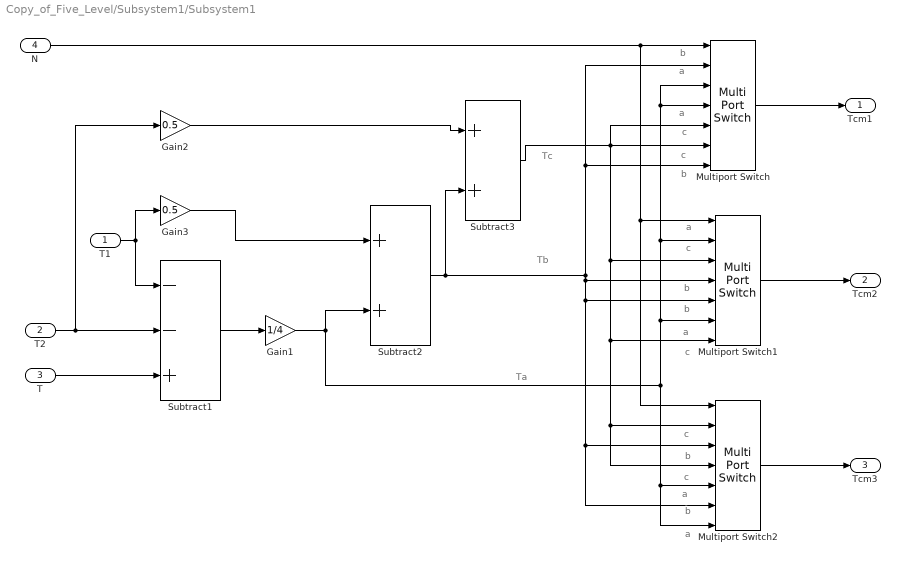
== system Copy_of_Five_Level/Subsystem1/Subsystem1 ==
  note: Ta
  note: Tb
  note: Tc
  note: b
  note: a
  note: a
  note: c
  note: c
  note: b
  note: a
  note: c
  note: b
  note: b
  note: a
  note: c
  note: c
  note: b
  note: c
  note: a
  note: b
  note: a
  T1 : Inport
  T2 : Inport  Port=2
  T : Inport  Port=3
  N : Inport  Port=4
  Gain1 : Gain  Gain=1/4
  Gain2 : Gain  Gain=0.5
  Gain3 : Gain  Gain=0.5
  Multiport Switch : MultiPortSwitch  Inputs=6
  Multiport Switch1 : MultiPortSwitch  Inputs=6
  Multiport Switch2 : MultiPortSwitch  Inputs=6
  Subtract1 : Sum  Inputs=--+
  Subtract2 : Sum
  Subtract3 : Sum
  Tcm1 : Outport
  Tcm2 : Outport  Port=2
  Tcm3 : Outport  Port=3
  wires:
  T2/1 -> Gain2/1, Subtract1/2
  T/1 -> Subtract1/3
  T1/1 -> Gain3/1, Subtract1/1
  Gain3/1 -> Subtract2/1
  Subtract1/1 -> Gain1/1
  Gain1/1 -> Subtract2/2, Multiport Switch/3, Multiport Switch/4, Multiport Switch1/2, Multiport Switch1/6, Multiport Switch2/5, Multiport Switch2/7
  Subtract2/1 -> Subtract3/2, Multiport Switch/2, Multiport Switch/7, Multiport Switch1/4, Multiport Switch1/5, Multiport Switch2/3, Multiport Switch2/6
  Gain2/1 -> Subtract3/1
  N/1 -> Multiport Switch/1, Multiport Switch2/1, Multiport Switch1/1
  Multiport Switch/1 -> Tcm1/1
  Multiport Switch1/1 -> Tcm2/1
  Multiport Switch2/1 -> Tcm3/1
  Subtract3/1 -> Multiport Switch/5, Multiport Switch/6, Multiport Switch1/3, Multiport Switch1/7, Multiport Switch2/2, Multiport Switch2/4

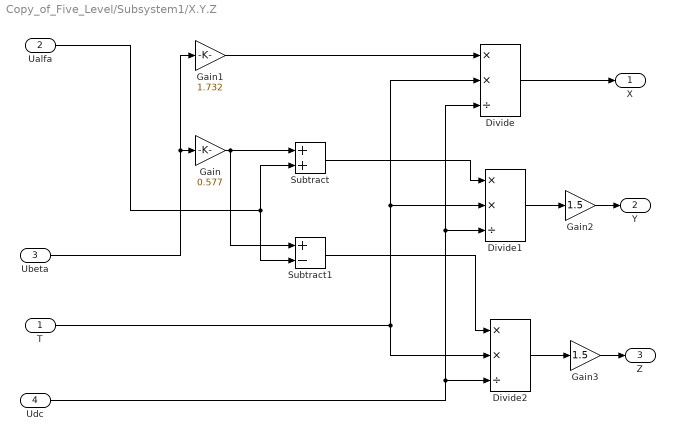
== system Copy_of_Five_Level/Subsystem1/X.Y.Z ==
  T : Inport
  Ualfa : Inport  Port=2
  Ubeta : Inport  Port=3
  Udc : Inport  Port=4
  Divide : Product  Inputs=**/
  Divide1 : Product  Inputs=**/
  Divide2 : Product  Inputs=**/
  Gain : Gain  Gain=0.577
  Gain1 : Gain  Gain=1.732
  Gain2 : Gain  Gain=1.5
  Gain3 : Gain  Gain=1.5
  Subtract : Sum
  Subtract1 : Sum  Inputs=+-
  X : Outport
  Y : Outport  Port=2
  Z : Outport  Port=3
  wires:
  Gain/1 -> Subtract/1, Subtract1/1
  Gain1/1 -> Divide/1
  T/1 -> Divide2/2, Divide1/2, Divide/2
  Udc/1 -> Divide2/3, Divide1/3, Divide/3
  Ualfa/1 -> Subtract1/2, Subtract/2
  Subtract/1 -> Divide1/1
  Subtract1/1 -> Divide2/1
  Divide/1 -> X/1
  Divide1/1 -> Gain2/1
  Divide2/1 -> Gain3/1
  Gain2/1 -> Y/1
  Gain3/1 -> Z/1
  Ubeta/1 -> Gain1/1, Gain/1

== system Copy_of_Five_Level/bridge1/T1 ==
  G : Inport
  D1 : powerlib/Power Electronics/Diode  Ron=0.001  Lon=0  Vf=0.8  IC=0  UseSnubber=off  Rs=1e6  Cs=250e-9  Measurements=off
  S1 : powerlib/Power Electronics/Ideal Switch  Ron=0.001  Lon=0  IC=0  Rs=inf  Cs=0  Measurements=on
  C : PMIOPort  Port=1  Side=Left
  E : PMIOPort  Port=2  Side=Right
  m : Outport
  wires:
  S1/1 -> m/1
  G/1 -> S1/1
  connections:
  D1/LConn1 -- S1/LConn1 -- E/RConn1
  D1/RConn1 -- S1/RConn1 -- C/RConn1

== system Copy_of_Five_Level/bridge1/T10 ==
  G : Inport
  D1 : powerlib/Power Electronics/Diode  Ron=0.001  Lon=0  Vf=0.8  IC=0  UseSnubber=off  Rs=1e6  Cs=250e-9  Measurements=off
  S1 : powerlib/Power Electronics/Ideal Switch  Ron=0.001  Lon=0  IC=0  Rs=inf  Cs=0  Measurements=on
  C : PMIOPort  Port=1  Side=Left
  E : PMIOPort  Port=2  Side=Right
  m : Outport
  wires:
  S1/1 -> m/1
  G/1 -> S1/1
  connections:
  D1/LConn1 -- S1/LConn1 -- E/RConn1
  D1/RConn1 -- S1/RConn1 -- C/RConn1

== system Copy_of_Five_Level/bridge1/T2 ==
  G : Inport
  D1 : powerlib/Power Electronics/Diode  Ron=0.001  Lon=0  Vf=0.8  IC=0  UseSnubber=off  Rs=1e6  Cs=250e-9  Measurements=off
  S1 : powerlib/Power Electronics/Ideal Switch  Ron=0.001  Lon=0  IC=0  Rs=inf  Cs=0  Measurements=on
  C : PMIOPort  Port=1  Side=Left
  E : PMIOPort  Port=2  Side=Right
  m : Outport
  wires:
  S1/1 -> m/1
  G/1 -> S1/1
  connections:
  D1/LConn1 -- S1/LConn1 -- E/RConn1
  D1/RConn1 -- S1/RConn1 -- C/RConn1

== system Copy_of_Five_Level/bridge1/T3 ==
  G : Inport
  D1 : powerlib/Power Electronics/Diode  Ron=0.001  Lon=0  Vf=0.8  IC=0  UseSnubber=off  Rs=1e6  Cs=250e-9  Measurements=off
  S1 : powerlib/Power Electronics/Ideal Switch  Ron=0.001  Lon=0  IC=0  Rs=inf  Cs=0  Measurements=on
  C : PMIOPort  Port=1  Side=Left
  E : PMIOPort  Port=2  Side=Right
  m : Outport
  wires:
  S1/1 -> m/1
  G/1 -> S1/1
  connections:
  D1/LConn1 -- S1/LConn1 -- E/RConn1
  D1/RConn1 -- S1/RConn1 -- C/RConn1

== system Copy_of_Five_Level/bridge1/T4 ==
  G : Inport
  D1 : powerlib/Power Electronics/Diode  Ron=0.001  Lon=0  Vf=0.8  IC=0  UseSnubber=off  Rs=1e6  Cs=250e-9  Measurements=off
  S1 : powerlib/Power Electronics/Ideal Switch  Ron=0.001  Lon=0  IC=0  Rs=inf  Cs=0  Measurements=on
  C : PMIOPort  Port=1  Side=Left
  E : PMIOPort  Port=2  Side=Right
  m : Outport
  wires:
  S1/1 -> m/1
  G/1 -> S1/1
  connections:
  D1/LConn1 -- S1/LConn1 -- E/RConn1
  D1/RConn1 -- S1/RConn1 -- C/RConn1

== system Copy_of_Five_Level/bridge1/T5 ==
  G : Inport
  D1 : powerlib/Power Electronics/Diode  Ron=0.001  Lon=0  Vf=0.8  IC=0  UseSnubber=off  Rs=1e6  Cs=250e-9  Measurements=off
  S1 : powerlib/Power Electronics/Ideal Switch  Ron=0.001  Lon=0  IC=0  Rs=inf  Cs=0  Measurements=on
  C : PMIOPort  Port=1  Side=Left
  E : PMIOPort  Port=2  Side=Right
  m : Outport
  wires:
  S1/1 -> m/1
  G/1 -> S1/1
  connections:
  D1/LConn1 -- S1/LConn1 -- E/RConn1
  D1/RConn1 -- S1/RConn1 -- C/RConn1

== system Copy_of_Five_Level/bridge1/T6 ==
  G : Inport
  D1 : powerlib/Power Electronics/Diode  Ron=0.001  Lon=0  Vf=0.8  IC=0  UseSnubber=off  Rs=1e6  Cs=250e-9  Measurements=off
  S1 : powerlib/Power Electronics/Ideal Switch  Ron=0.001  Lon=0  IC=0  Rs=inf  Cs=0  Measurements=on
  C : PMIOPort  Port=1  Side=Left
  E : PMIOPort  Port=2  Side=Right
  m : Outport
  wires:
  S1/1 -> m/1
  G/1 -> S1/1
  connections:
  D1/LConn1 -- S1/LConn1 -- E/RConn1
  D1/RConn1 -- S1/RConn1 -- C/RConn1

== system Copy_of_Five_Level/bridge1/T7 ==
  G : Inport
  D1 : powerlib/Power Electronics/Diode  Ron=0.001  Lon=0  Vf=0.8  IC=0  UseSnubber=off  Rs=1e6  Cs=250e-9  Measurements=off
  S1 : powerlib/Power Electronics/Ideal Switch  Ron=0.001  Lon=0  IC=0  Rs=inf  Cs=0  Measurements=on
  C : PMIOPort  Port=1  Side=Left
  E : PMIOPort  Port=2  Side=Right
  m : Outport
  wires:
  S1/1 -> m/1
  G/1 -> S1/1
  connections:
  D1/LConn1 -- S1/LConn1 -- E/RConn1
  D1/RConn1 -- S1/RConn1 -- C/RConn1

== system Copy_of_Five_Level/bridge1/T8 ==
  G : Inport
  D1 : powerlib/Power Electronics/Diode  Ron=0.001  Lon=0  Vf=0.8  IC=0  UseSnubber=off  Rs=1e6  Cs=250e-9  Measurements=off
  S1 : powerlib/Power Electronics/Ideal Switch  Ron=0.001  Lon=0  IC=0  Rs=inf  Cs=0  Measurements=on
  C : PMIOPort  Port=1  Side=Left
  E : PMIOPort  Port=2  Side=Right
  m : Outport
  wires:
  S1/1 -> m/1
  G/1 -> S1/1
  connections:
  D1/LConn1 -- S1/LConn1 -- E/RConn1
  D1/RConn1 -- S1/RConn1 -- C/RConn1

== system Copy_of_Five_Level/bridge1/T9 ==
  G : Inport
  D1 : powerlib/Power Electronics/Diode  Ron=0.001  Lon=0  Vf=0.8  IC=0  UseSnubber=off  Rs=1e6  Cs=250e-9  Measurements=off
  S1 : powerlib/Power Electronics/Ideal Switch  Ron=0.001  Lon=0  IC=0  Rs=inf  Cs=0  Measurements=on
  C : PMIOPort  Port=1  Side=Left
  E : PMIOPort  Port=2  Side=Right
  m : Outport
  wires:
  S1/1 -> m/1
  G/1 -> S1/1
  connections:
  D1/LConn1 -- S1/LConn1 -- E/RConn1
  D1/RConn1 -- S1/RConn1 -- C/RConn1

== system Copy_of_Five_Level/bridge2/T1 ==
  G : Inport
  D1 : powerlib/Power Electronics/Diode  Ron=0.001  Lon=0  Vf=0.8  IC=0  UseSnubber=off  Rs=1e6  Cs=250e-9  Measurements=off
  S1 : powerlib/Power Electronics/Ideal Switch  Ron=0.001  Lon=0  IC=0  Rs=inf  Cs=0  Measurements=on
  C : PMIOPort  Port=1  Side=Left
  E : PMIOPort  Port=2  Side=Right
  m : Outport
  wires:
  S1/1 -> m/1
  G/1 -> S1/1
  connections:
  D1/LConn1 -- S1/LConn1 -- E/RConn1
  D1/RConn1 -- S1/RConn1 -- C/RConn1

== system Copy_of_Five_Level/bridge2/T10 ==
  G : Inport
  D1 : powerlib/Power Electronics/Diode  Ron=0.001  Lon=0  Vf=0.8  IC=0  UseSnubber=off  Rs=1e6  Cs=250e-9  Measurements=off
  S1 : powerlib/Power Electronics/Ideal Switch  Ron=0.001  Lon=0  IC=0  Rs=inf  Cs=0  Measurements=on
  C : PMIOPort  Port=1  Side=Left
  E : PMIOPort  Port=2  Side=Right
  m : Outport
  wires:
  S1/1 -> m/1
  G/1 -> S1/1
  connections:
  D1/LConn1 -- S1/LConn1 -- E/RConn1
  D1/RConn1 -- S1/RConn1 -- C/RConn1

== system Copy_of_Five_Level/bridge2/T2 ==
  G : Inport
  D1 : powerlib/Power Electronics/Diode  Ron=0.001  Lon=0  Vf=0.8  IC=0  UseSnubber=off  Rs=1e6  Cs=250e-9  Measurements=off
  S1 : powerlib/Power Electronics/Ideal Switch  Ron=0.001  Lon=0  IC=0  Rs=inf  Cs=0  Measurements=on
  C : PMIOPort  Port=1  Side=Left
  E : PMIOPort  Port=2  Side=Right
  m : Outport
  wires:
  S1/1 -> m/1
  G/1 -> S1/1
  connections:
  D1/LConn1 -- S1/LConn1 -- E/RConn1
  D1/RConn1 -- S1/RConn1 -- C/RConn1

== system Copy_of_Five_Level/bridge2/T3 ==
  G : Inport
  D1 : powerlib/Power Electronics/Diode  Ron=0.001  Lon=0  Vf=0.8  IC=0  UseSnubber=off  Rs=1e6  Cs=250e-9  Measurements=off
  S1 : powerlib/Power Electronics/Ideal Switch  Ron=0.001  Lon=0  IC=0  Rs=inf  Cs=0  Measurements=on
  C : PMIOPort  Port=1  Side=Left
  E : PMIOPort  Port=2  Side=Right
  m : Outport
  wires:
  S1/1 -> m/1
  G/1 -> S1/1
  connections:
  D1/LConn1 -- S1/LConn1 -- E/RConn1
  D1/RConn1 -- S1/RConn1 -- C/RConn1

== system Copy_of_Five_Level/bridge2/T4 ==
  G : Inport
  D1 : powerlib/Power Electronics/Diode  Ron=0.001  Lon=0  Vf=0.8  IC=0  UseSnubber=off  Rs=1e6  Cs=250e-9  Measurements=off
  S1 : powerlib/Power Electronics/Ideal Switch  Ron=0.001  Lon=0  IC=0  Rs=inf  Cs=0  Measurements=on
  C : PMIOPort  Port=1  Side=Left
  E : PMIOPort  Port=2  Side=Right
  m : Outport
  wires:
  S1/1 -> m/1
  G/1 -> S1/1
  connections:
  D1/LConn1 -- S1/LConn1 -- E/RConn1
  D1/RConn1 -- S1/RConn1 -- C/RConn1

== system Copy_of_Five_Level/bridge2/T5 ==
  G : Inport
  D1 : powerlib/Power Electronics/Diode  Ron=0.001  Lon=0  Vf=0.8  IC=0  UseSnubber=off  Rs=1e6  Cs=250e-9  Measurements=off
  S1 : powerlib/Power Electronics/Ideal Switch  Ron=0.001  Lon=0  IC=0  Rs=inf  Cs=0  Measurements=on
  C : PMIOPort  Port=1  Side=Left
  E : PMIOPort  Port=2  Side=Right
  m : Outport
  wires:
  S1/1 -> m/1
  G/1 -> S1/1
  connections:
  D1/LConn1 -- S1/LConn1 -- E/RConn1
  D1/RConn1 -- S1/RConn1 -- C/RConn1

== system Copy_of_Five_Level/bridge2/T6 ==
  G : Inport
  D1 : powerlib/Power Electronics/Diode  Ron=0.001  Lon=0  Vf=0.8  IC=0  UseSnubber=off  Rs=1e6  Cs=250e-9  Measurements=off
  S1 : powerlib/Power Electronics/Ideal Switch  Ron=0.001  Lon=0  IC=0  Rs=inf  Cs=0  Measurements=on
  C : PMIOPort  Port=1  Side=Left
  E : PMIOPort  Port=2  Side=Right
  m : Outport
  wires:
  S1/1 -> m/1
  G/1 -> S1/1
  connections:
  D1/LConn1 -- S1/LConn1 -- E/RConn1
  D1/RConn1 -- S1/RConn1 -- C/RConn1

== system Copy_of_Five_Level/bridge2/T7 ==
  G : Inport
  D1 : powerlib/Power Electronics/Diode  Ron=0.001  Lon=0  Vf=0.8  IC=0  UseSnubber=off  Rs=1e6  Cs=250e-9  Measurements=off
  S1 : powerlib/Power Electronics/Ideal Switch  Ron=0.001  Lon=0  IC=0  Rs=inf  Cs=0  Measurements=on
  C : PMIOPort  Port=1  Side=Left
  E : PMIOPort  Port=2  Side=Right
  m : Outport
  wires:
  S1/1 -> m/1
  G/1 -> S1/1
  connections:
  D1/LConn1 -- S1/LConn1 -- E/RConn1
  D1/RConn1 -- S1/RConn1 -- C/RConn1

== system Copy_of_Five_Level/bridge2/T8 ==
  G : Inport
  D1 : powerlib/Power Electronics/Diode  Ron=0.001  Lon=0  Vf=0.8  IC=0  UseSnubber=off  Rs=1e6  Cs=250e-9  Measurements=off
  S1 : powerlib/Power Electronics/Ideal Switch  Ron=0.001  Lon=0  IC=0  Rs=inf  Cs=0  Measurements=on
  C : PMIOPort  Port=1  Side=Left
  E : PMIOPort  Port=2  Side=Right
  m : Outport
  wires:
  S1/1 -> m/1
  G/1 -> S1/1
  connections:
  D1/LConn1 -- S1/LConn1 -- E/RConn1
  D1/RConn1 -- S1/RConn1 -- C/RConn1

== system Copy_of_Five_Level/bridge2/T9 ==
  G : Inport
  D1 : powerlib/Power Electronics/Diode  Ron=0.001  Lon=0  Vf=0.8  IC=0  UseSnubber=off  Rs=1e6  Cs=250e-9  Measurements=off
  S1 : powerlib/Power Electronics/Ideal Switch  Ron=0.001  Lon=0  IC=0  Rs=inf  Cs=0  Measurements=on
  C : PMIOPort  Port=1  Side=Left
  E : PMIOPort  Port=2  Side=Right
  m : Outport
  wires:
  S1/1 -> m/1
  G/1 -> S1/1
  connections:
  D1/LConn1 -- S1/LConn1 -- E/RConn1
  D1/RConn1 -- S1/RConn1 -- C/RConn1

== system Copy_of_Five_Level/bridge3/T1 ==
  G : Inport
  D1 : powerlib/Power Electronics/Diode  Ron=0.001  Lon=0  Vf=0.8  IC=0  UseSnubber=off  Rs=1e6  Cs=250e-9  Measurements=off
  S1 : powerlib/Power Electronics/Ideal Switch  Ron=0.001  Lon=0  IC=0  Rs=inf  Cs=0  Measurements=on
  C : PMIOPort  Port=1  Side=Left
  E : PMIOPort  Port=2  Side=Right
  m : Outport
  wires:
  S1/1 -> m/1
  G/1 -> S1/1
  connections:
  D1/LConn1 -- S1/LConn1 -- E/RConn1
  D1/RConn1 -- S1/RConn1 -- C/RConn1

== system Copy_of_Five_Level/bridge3/T10 ==
  G : Inport
  D1 : powerlib/Power Electronics/Diode  Ron=0.001  Lon=0  Vf=0.8  IC=0  UseSnubber=off  Rs=1e6  Cs=250e-9  Measurements=off
  S1 : powerlib/Power Electronics/Ideal Switch  Ron=0.001  Lon=0  IC=0  Rs=inf  Cs=0  Measurements=on
  C : PMIOPort  Port=1  Side=Left
  E : PMIOPort  Port=2  Side=Right
  m : Outport
  wires:
  S1/1 -> m/1
  G/1 -> S1/1
  connections:
  D1/LConn1 -- S1/LConn1 -- E/RConn1
  D1/RConn1 -- S1/RConn1 -- C/RConn1

== system Copy_of_Five_Level/bridge3/T2 ==
  G : Inport
  D1 : powerlib/Power Electronics/Diode  Ron=0.001  Lon=0  Vf=0.8  IC=0  UseSnubber=off  Rs=1e6  Cs=250e-9  Measurements=off
  S1 : powerlib/Power Electronics/Ideal Switch  Ron=0.001  Lon=0  IC=0  Rs=inf  Cs=0  Measurements=on
  C : PMIOPort  Port=1  Side=Left
  E : PMIOPort  Port=2  Side=Right
  m : Outport
  wires:
  S1/1 -> m/1
  G/1 -> S1/1
  connections:
  D1/LConn1 -- S1/LConn1 -- E/RConn1
  D1/RConn1 -- S1/RConn1 -- C/RConn1

== system Copy_of_Five_Level/bridge3/T3 ==
  G : Inport
  D1 : powerlib/Power Electronics/Diode  Ron=0.001  Lon=0  Vf=0.8  IC=0  UseSnubber=off  Rs=1e6  Cs=250e-9  Measurements=off
  S1 : powerlib/Power Electronics/Ideal Switch  Ron=0.001  Lon=0  IC=0  Rs=inf  Cs=0  Measurements=on
  C : PMIOPort  Port=1  Side=Left
  E : PMIOPort  Port=2  Side=Right
  m : Outport
  wires:
  S1/1 -> m/1
  G/1 -> S1/1
  connections:
  D1/LConn1 -- S1/LConn1 -- E/RConn1
  D1/RConn1 -- S1/RConn1 -- C/RConn1

== system Copy_of_Five_Level/bridge3/T4 ==
  G : Inport
  D1 : powerlib/Power Electronics/Diode  Ron=0.001  Lon=0  Vf=0.8  IC=0  UseSnubber=off  Rs=1e6  Cs=250e-9  Measurements=off
  S1 : powerlib/Power Electronics/Ideal Switch  Ron=0.001  Lon=0  IC=0  Rs=inf  Cs=0  Measurements=on
  C : PMIOPort  Port=1  Side=Left
  E : PMIOPort  Port=2  Side=Right
  m : Outport
  wires:
  S1/1 -> m/1
  G/1 -> S1/1
  connections:
  D1/LConn1 -- S1/LConn1 -- E/RConn1
  D1/RConn1 -- S1/RConn1 -- C/RConn1

== system Copy_of_Five_Level/bridge3/T5 ==
  G : Inport
  D1 : powerlib/Power Electronics/Diode  Ron=0.001  Lon=0  Vf=0.8  IC=0  UseSnubber=off  Rs=1e6  Cs=250e-9  Measurements=off
  S1 : powerlib/Power Electronics/Ideal Switch  Ron=0.001  Lon=0  IC=0  Rs=inf  Cs=0  Measurements=on
  C : PMIOPort  Port=1  Side=Left
  E : PMIOPort  Port=2  Side=Right
  m : Outport
  wires:
  S1/1 -> m/1
  G/1 -> S1/1
  connections:
  D1/LConn1 -- S1/LConn1 -- E/RConn1
  D1/RConn1 -- S1/RConn1 -- C/RConn1

== system Copy_of_Five_Level/bridge3/T6 ==
  G : Inport
  D1 : powerlib/Power Electronics/Diode  Ron=0.001  Lon=0  Vf=0.8  IC=0  UseSnubber=off  Rs=1e6  Cs=250e-9  Measurements=off
  S1 : powerlib/Power Electronics/Ideal Switch  Ron=0.001  Lon=0  IC=0  Rs=inf  Cs=0  Measurements=on
  C : PMIOPort  Port=1  Side=Left
  E : PMIOPort  Port=2  Side=Right
  m : Outport
  wires:
  S1/1 -> m/1
  G/1 -> S1/1
  connections:
  D1/LConn1 -- S1/LConn1 -- E/RConn1
  D1/RConn1 -- S1/RConn1 -- C/RConn1

== system Copy_of_Five_Level/bridge3/T7 ==
  G : Inport
  D1 : powerlib/Power Electronics/Diode  Ron=0.001  Lon=0  Vf=0.8  IC=0  UseSnubber=off  Rs=1e6  Cs=250e-9  Measurements=off
  S1 : powerlib/Power Electronics/Ideal Switch  Ron=0.001  Lon=0  IC=0  Rs=inf  Cs=0  Measurements=on
  C : PMIOPort  Port=1  Side=Left
  E : PMIOPort  Port=2  Side=Right
  m : Outport
  wires:
  S1/1 -> m/1
  G/1 -> S1/1
  connections:
  D1/LConn1 -- S1/LConn1 -- E/RConn1
  D1/RConn1 -- S1/RConn1 -- C/RConn1

== system Copy_of_Five_Level/bridge3/T8 ==
  G : Inport
  D1 : powerlib/Power Electronics/Diode  Ron=0.001  Lon=0  Vf=0.8  IC=0  UseSnubber=off  Rs=1e6  Cs=250e-9  Measurements=off
  S1 : powerlib/Power Electronics/Ideal Switch  Ron=0.001  Lon=0  IC=0  Rs=inf  Cs=0  Measurements=on
  C : PMIOPort  Port=1  Side=Left
  E : PMIOPort  Port=2  Side=Right
  m : Outport
  wires:
  S1/1 -> m/1
  G/1 -> S1/1
  connections:
  D1/LConn1 -- S1/LConn1 -- E/RConn1
  D1/RConn1 -- S1/RConn1 -- C/RConn1

== system Copy_of_Five_Level/bridge3/T9 ==
  G : Inport
  D1 : powerlib/Power Electronics/Diode  Ron=0.001  Lon=0  Vf=0.8  IC=0  UseSnubber=off  Rs=1e6  Cs=250e-9  Measurements=off
  S1 : powerlib/Power Electronics/Ideal Switch  Ron=0.001  Lon=0  IC=0  Rs=inf  Cs=0  Measurements=on
  C : PMIOPort  Port=1  Side=Left
  E : PMIOPort  Port=2  Side=Right
  m : Outport
  wires:
  S1/1 -> m/1
  G/1 -> S1/1
  connections:
  D1/LConn1 -- S1/LConn1 -- E/RConn1
  D1/RConn1 -- S1/RConn1 -- C/RConn1
